simulink model "Smith_Predictor"  (R2019b)
settings: Solver=ode45  StartTime=0.0  StopTime=10.0  FixedStep=0.001  RelTol=1e-5  AbsTol=1e-5
settings Model: Creator=meetn  LastModifiedBy=manth

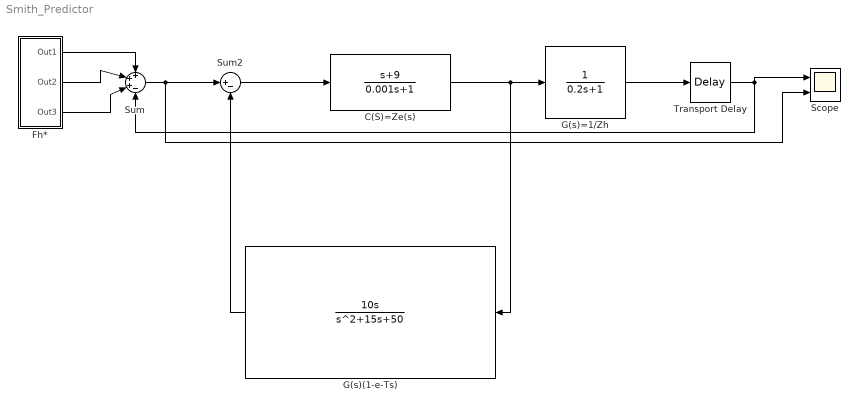
== system Smith_Predictor ==
  C(S)=Ze(s) : TransferFcn  Numerator=[1 9]  Denominator=[0.001 1]
  Fh* : Subsystem
  G(s)(1-e-Ts) : TransferFcn  Numerator=[10 0]  Denominator=[1 15 50]
  G(s)=1/Zh : TransferFcn  Denominator=[0.2 1]
  Scope : Scope  NumInputPorts=2
  Sum : Sum  Inputs=+++-
  Sum2 : Sum  Inputs=|+-
  Transport Delay : TransportDelay  DelayTime=0.1
  wires:
  Sum/1 -> Scope/2, Sum2/1
  Sum2/1 -> C(S)=Ze(s)/1
  C(S)=Ze(s)/1 -> G(s)(1-e-Ts)/1, G(s)=1/Zh/1
  G(s)=1/Zh/1 -> Transport Delay/1
  G(s)(1-e-Ts)/1 -> Sum2/2
  Transport Delay/1 -> Scope/1, Sum/4
  Fh*/1(Out1) -> Sum/1
  Fh*/2(Out2) -> Sum/2
  Fh*/3(Out3) -> Sum/3

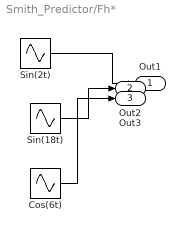
== system Smith_Predictor/Fh* ==
  Cos(6t) : Sin  Frequency=6  Phase=pi/2  SampleTime=0
  Sin(18t) : Sin  Frequency=18  SampleTime=0
  Sin(2t) : Sin  Frequency=2  SampleTime=0
  Out1 : Outport
  Out2 : Outport  Port=2
  Out3 : Outport  Port=3
  wires:
  Sin(18t)/1 -> Out2/1
  Sin(2t)/1 -> Out1/1
  Cos(6t)/1 -> Out3/1
